simulink model "pendulum_demo"  (Simulink 6.0)
settings: Solver=ode45  SolverMode=SingleTasking  StartTime=0  StopTime=15  RelTol=1e-3  AbsTol=1e-6
PreLoadFcn:
  | load pendulum_demo
undefined symbols (not defined in the file or in its folder): Kf, Ki, Klqr, Kp
libraries: srolib x2
settings Model: Creator=pascal  LastModifiedBy=pascal  ExtModeTrigMode=oneshot
settings DataIOCC: LimitDataPoints=off  SaveOutput=off  SaveTime=off  SignalLoggingName=logsOut
settings OptimizationCC: BooleanDataType=off
settings DebuggingCC: ConsistencyChecking=warning  CheckExecutionContextPreStartOutputMsg=on  CheckExecutionContextRuntimeOutputMsg=on  SolverPrmCheckMsg=none
settings HardwareCC: TargetUnknown=on
settings ModelReferenceCC: UpdateModelReferenceTargets=IfOutOfDate
settings RTWCC: TemplateMakefile=grt_vc.tmf
settings SFSimCC: SFSimApplyToAllLibs=on  SFSimBuildMode=Incremental

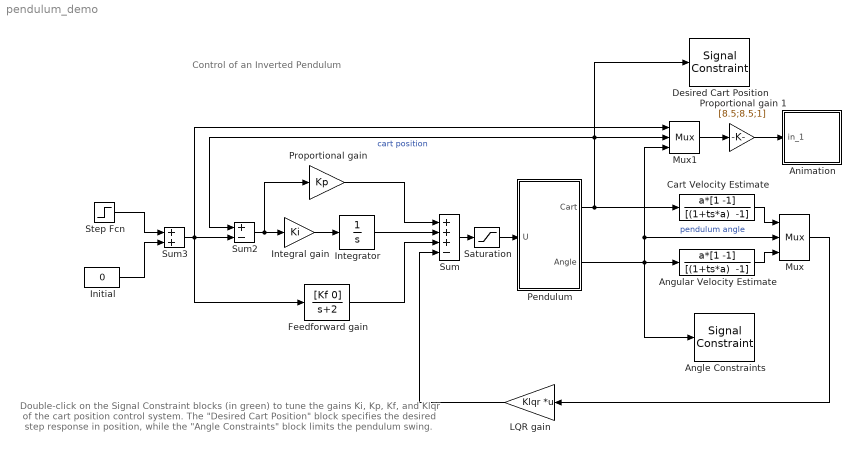
== system pendulum_demo ==
  note: Control of an Inverted Pendulum
  note: Double-click on the Signal Constraint blocks (in green)
      | to tune the gains Ki, Kp, Kf, and Klqr of
      | the cart position control system.
      |
      | The "Desired Cart Position" block specifies the desired
      | step response in position, while the "Angle Constraints"
      | block limits the pendulum swing.
  Angle Constraints : srolib/Signal Constraint  DialogPosition=[0.2825 0.305 0.263125 0.2475]  SaveIn=workspace  SaveAs=pendulum_optim  LogID=SRO_DataLog_1
  Angular Velocity Estimate : DiscreteTransferFcn  Numerator=a*[1 -1]  Denominator="[(1+ts*a)  -1]"  SampleTime=ts  mask(Finite difference velocity estimator with filter.){@1=10, @2=0.01}
      mask prompts: @1 "Cutoff frequency( hz ):"; @2 "Sample time:"
      mask help: Finite difference velocity estimator with filter.
      mask init:
      | hz =@1; a=hz*2*pi; ts=@2;
      mask Display: disp('FD w/ filter')
  Animation : Subsystem  PropExecContextAcrossSSBoundary=on  mask(Pendulum plot){@1=Initial}
      mask prompts: @1 "DC reference signal block name:"
      mask help: Pendulum plot
      mask init:
      | RefBlock=&1;
      mask Help: Pendulum animation function using Handle graphics.
      mask Display: plot([-10 10],[0 0],[-2 -2 2 2],[0 1 1 0],[0 3],[1 5])
  Cart Velocity Estimate : DiscreteTransferFcn  Numerator=a*[1 -1]  Denominator="[(1+ts*a)  -1]"  SampleTime=ts  mask(Finite difference velocity estimator with filter.){@1=10, @2=0.01}
      mask prompts: @1 "Cutoff frequency( hz ):"; @2 "Sample time:"
      mask help: Finite difference velocity estimator with filter.
      mask init:
      | hz =@1; a=hz*2*pi; ts=@2;
      mask Display: disp('FD w/ filter')
  Desired Cart Position : srolib/Signal Constraint  DialogPosition=[0.01125 0.305 0.265625 0.2475]  SaveIn=workspace  SaveAs=pendulum_optim  LogID=SRO_DataLog_2
  Feedforward gain : TransferFcn  Numerator=[Kf 0]  Denominator=[1 2]
  Initial : Constant  Value=0
  Integral gain : Gain  Gain=Ki  SaturateOnIntegerOverflow=on
  Integrator : Integrator  LimitOutput=on  UpperSaturationLimit=5  LowerSaturationLimit=-5
  LQR gain : Gain  Orientation=left  Gain=Klqr  Multiplication=Matrix(K*u)
  Mux : Mux  Inputs=3
  Mux1 : Mux  Inputs=3
  Pendulum : Subsystem  PropExecContextAcrossSSBoundary=on  mask(Inverted pendulum on cart){@1=0.455, @2=0.21, @3=0.61/2, @4=9.8}
      mask prompts: @1 "Mass of cart (kg):"; @2 "Mass of pendulum (kg):"; @3 "Distance to pendulum center of mass(m):"; @4 "Acceleration of gravity (m/s^2):"
      mask help: Unmask and double-click to see dynamics
      mask init:
      | M=@1; m=@2; l=@3; g=@4;
      mask Help: Nonlinear dynamics of inverted pendulum on cart.
  "Proportional gain " : Gain  Gain=Kp  SaturateOnIntegerOverflow=on
  Proportional gain 1 : Gain  Gain=[8.5;8.5;1]  SaturateOnIntegerOverflow=on
  Saturation : Saturate  UpperLimit=1  LowerLimit=-1
  Step Fcn : Step  Time=0  SampleTime=0
  Sum : Sum  Inputs=+++-  SaturateOnIntegerOverflow=on  InputSameDT=on
  Sum2 : Sum  Inputs=+-  SaturateOnIntegerOverflow=on  InputSameDT=on
  Sum3 : Sum  SaturateOnIntegerOverflow=on  InputSameDT=on
  wires:
  Mux/1 -> LQR gain/1
  LQR gain/1 -> Sum/4
  Sum2/1 -> Integral gain/1, "Proportional gain "/1
  Integral gain/1 -> Integrator/1
  Sum/1 -> Saturation/1
  "Proportional gain "/1 -> Sum/1
  Feedforward gain/1 -> Sum/3
  Sum3/1 -> Feedforward gain/1, Sum2/2, Mux1/1
  Integrator/1 -> Sum/2
  Saturation/1 -> Pendulum/1(U)
  Pendulum/1(Cart) -> Sum2/1, Desired Cart Position/1, Mux1/2, Cart Velocity Estimate/1  "cart position"
  Cart Velocity Estimate/1 -> Mux/1
  Angular Velocity Estimate/1 -> Mux/3
  Mux1/1 -> Proportional gain 1/1
  Initial/1 -> Sum3/2
  Step Fcn/1 -> Sum3/1
  Pendulum/2(Angle) -> Angular Velocity Estimate/1, Angle Constraints/1, Mux1/3, Mux/2  "pendulum angle"
  Proportional gain 1/1 -> Animation/1(in_1)

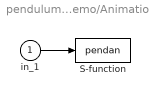
== system pendulum_demo/Animation ==
  in_1 : Inport  LatchInput=off
  S-function : S-Function  FunctionName=pendan  Parameters=RefBlock
      settings: DeleteFcn=pendan([],[],[],'DeleteBlock');
  wires:
  in_1/1 -> S-function/1

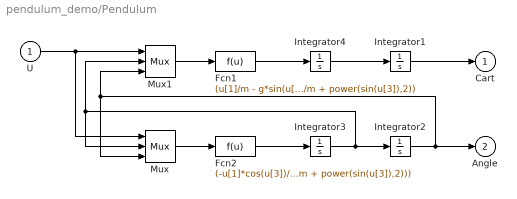
== system pendulum_demo/Pendulum ==
  U : Inport  LatchInput=off
  Fcn1 : Fcn  Expr=(u[1]/m - g*sin(u[3])*cos(u[3]) + l*power(u[2],2)*sin(u[3]))/(M/m + power(sin(u[3]),2))
  Fcn2 : Fcn  Expr=(-u[1]*cos(u[3])/m + (M+m)*g*sin(u[3])/m - l*power(u[2],2)*sin(u[3])*cos(u[3]))/(l*(M/m + power(sin(u[3]),2)))
  Integrator{1..4} (4 alike) : Integrator
  Mux : Mux  Inputs=3
  Mux1 : Mux  Inputs=3
  Cart : Outport  InitialOutput=0
  Angle : Outport  Port=2  InitialOutput=0
  wires:
  Integrator2/1 -> Mux/3, Mux1/3, Angle/1
  Integrator3/1 -> Mux/2, Mux1/2, Integrator2/1
  U/1 -> Mux/1, Mux1/1
  Integrator4/1 -> Integrator1/1
  Fcn1/1 -> Integrator4/1
  Mux1/1 -> Fcn1/1
  Mux/1 -> Fcn2/1
  Fcn2/1 -> Integrator3/1
  Integrator1/1 -> Cart/1
